simulink model "pitch_lin"  (R2017b)
settings: Solver=VariableStepAuto  StartTime=0.0  StopTime=10.0  RelTol=1e-3
values from neighbouring files (symbols this model uses):
  wb = .6    (= 0.6)    [Quad_vis.m]    (also in Sim_Constants.m; startup.m)
libraries: simulink x1, simulink_extras x1
settings Model: Creator=schapman  LastModifiedBy=schapman

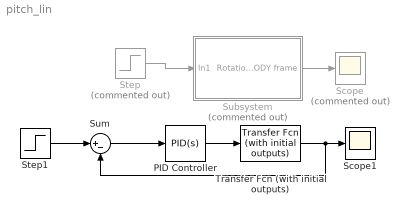
== system pitch_lin ==
  PID Controller : simulink/Continuous/PID Controller  Controller=PID  TimeDomain=Continuous-time  SampleTime=-1  IntegratorMethod=Forward Euler  FilterMethod=Forward Euler  Form=Parallel  UseFilter=on  ControllerParametersSource=internal  P=0.0586664338929351  I=0.00274645609516276  D=0.307715949952036  N=5.45397025421619  InitialConditionSource=internal  InitialConditionForIntegrator=0  InitialConditionForFilter=0  ExternalReset=none  LimitOutput=off  UpperSaturationLimit=inf  LowerSaturationLimit=-inf  LinearizeAsGain=on  AntiWindupMode=none  Kb=1  TrackingMode=off  Kt=1  PParamMin=[]  PParamMax=[]  IParamMin=[]  IParamMax=[]  DParamMin=[]  DParamMax=[]  NParamMin=[]  NParamMax=[]  KbParamMin=[]  KbParamMax=[]  KtParamMin=[]  KtParamMax=[]  POutMin=[]  POutMax=[]  IOutMin=[]  IOutMax=[]  DOutMin=[]  DOutMax=[]  NOutMin=[]  NOutMax=[]  KbOutMin=[]  KbOutMax=[]  KtOutMin=[]  KtOutMax=[]  IntegratorOutMin=[]  IntegratorOutMax=[]  FilterOutMin=[]  FilterOutMax=[]  SumOutMin=[]  SumOutMax=[]  SumI1OutMin=[]  SumI1OutMax=[]  SumI2OutMin=[]  SumI2OutMax=[]  SumI3OutMin=[]  SumI3OutMax=[]  SumDOutMin=[]  SumDOutMax=[]  SaturationOutMin=[]  SaturationOutMax=[]  IntegratorContinuousStateAttributes=''  IntegratorStateMustResolveToSignalObject=off  IntegratorRTWStateStorageClass=Auto  FilterContinuousStateAttributes=''  FilterStateMustResolveToSignalObject=off  FilterRTWStateStorageClass=Auto  DifferentiatorICPrevScaledInput=0  DifferentiatorOutMin=[]  DifferentiatorOutMax=[]  InitialConditionSetting=State (most efficient)  FilterDiffOutCoefMin=[]  FilterDiffOutCoefMax=[]  SumDenOutMin=[]  SumDenOutMax=[]  SumNumOutMin=[]  SumNumOutMax=[]  ReciprocalOutMin=[]  ReciprocalOutMax=[]  DivideOutMin=[]  DivideOutMax=[]  TunerSelectOption=Transfer Function Based (PID Tuner App)
  Scope : Scope  Commented=on
  Scope1 : Scope
  Step : Step  Commented=on  SampleTime=0
  Step1 : Step  SampleTime=0
  Subsystem : Subsystem  Commented=on
  Sum : Sum  Inputs=|+-
  Transfer Fcn (with initial outputs) : simulink_extras/Additional Linear/Transfer Fcn (with initial outputs)  N=[3.165]  D="[1  0 0 ]"  Y0=0  U0=0
  wires:
  Step/1 -> Subsystem/1(In1)
  Subsystem/1(Rotation in BODY frame) -> Scope/1
  PID Controller/1 -> Transfer Fcn (with initial outputs)/1
  Sum/1 -> PID Controller/1
  Transfer Fcn (with initial outputs)/1 -> Sum/2, Scope1/1
  Step1/1 -> Sum/1

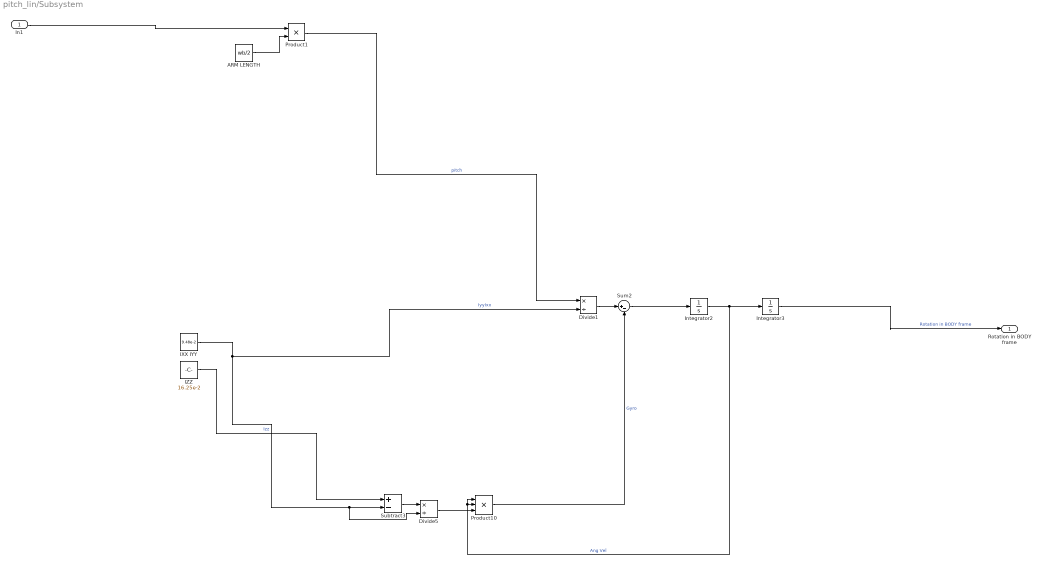
== system pitch_lin/Subsystem ==
  In1 : Inport
  ARM LENGTH : Constant  Value=wb/2
  Divide1 : Product  Inputs=*/
  Divide5 : Product  Inputs=*/
  IXX IYY : Constant  Value=9.48e-2
  IZZ : Constant  Value=16.25e-2
  Integrator2 : Integrator
  Integrator3 : Integrator
  Product1 : Product
  Product10 : Product  Inputs=3
  Subtract3 : Sum  Inputs=+-
  Sum2 : Sum  Inputs=|+-
  Rotation in BODY frame : Outport
  wires:
  Integrator2/1 -> Product10/2, Product10/1, Integrator3/1  "Ang Vel"
  IZZ/1 -> Subtract3/1  "Izz"
  IXX IYY/1 -> Divide1/2, Divide5/2, Subtract3/2  "IyyIxx"
  Divide5/1 -> Product10/3
  Subtract3/1 -> Divide5/1
  Divide1/1 -> Sum2/1
  Product10/1 -> Sum2/2  "Gyro"
  In1/1 -> Product1/1
  ARM LENGTH/1 -> Product1/2
  Product1/1 -> Divide1/1  "pitch"
  Sum2/1 -> Integrator2/1
  Integrator3/1 -> Rotation in BODY frame/1  "Rotation in BODY frame"
